simulink model "Joystick"  (R2023b)
settings: Solver=FixedStepAuto  StartTime=0.0  StopTime=t_Total  FixedStep=dt  RelTol=1e-3
undefined symbols (not defined in the file): delta_E_max, delta_E_min, delta_R_max, delta_R_min, dt
libraries: aerolibanimutils x2
settings Model: Creator=iwl  LastModifiedBy=iwl
settings ModelReferenceCC: EnableRefExpFcnMdlSchedulingChecks=on

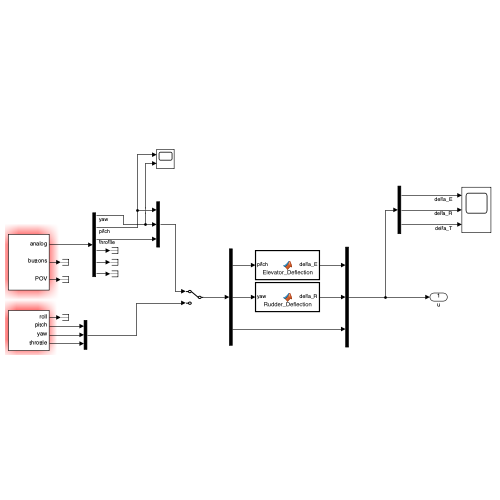
[thumbnail: Simulink's stored preview of the top-level diagram]
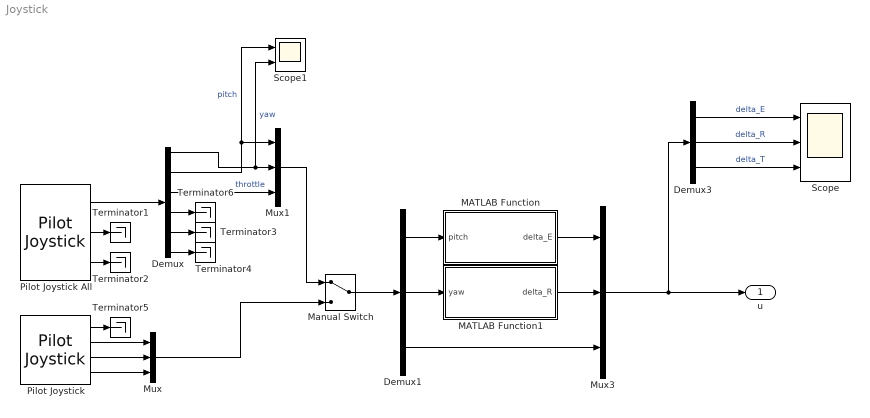
== system Joystick ==
  Demux : Demux  Outputs=6
  Demux1 : Demux  Outputs=3
  Demux3 : Demux  Outputs=3
  MATLAB Function : MATLAB Function  TreatAsAtomicUnit=on
  MATLAB Function1 : MATLAB Function  TreatAsAtomicUnit=on
  Manual Switch : ManualSwitch
  Mux : Mux  Inputs=3
  Mux1 : Mux  Inputs=3
  Mux3 : Mux  Inputs=3
  Pilot Joystick : aerolibanimutils/Pilot Joystick  JoystickID=Joystick1  OutputConfiguration=FourAxis  SampleTime=dt
  Pilot Joystick All : aerolibanimutils/Pilot Joystick  JoystickID=Joystick1  OutputConfiguration=AllOutputs  SampleTime=dt
  Scope : Scope  NumInputPorts=3
  Scope1 : Scope  NumInputPorts=2
  Terminator{1..6} (6 alike) : Terminator
  u : Outport
  wires:
  Pilot Joystick/1 -> Terminator5/1
  Demux/1 -> Scope1/2, Mux1/2  "yaw"
  Demux/5 -> Terminator3/1
  Mux1/1 -> Manual Switch/1
  Pilot Joystick All/1 -> Demux/1
  Mux/1 -> Manual Switch/2
  Demux1/3 -> Mux3/3
  Pilot Joystick All/2 -> Terminator1/1
  Pilot Joystick/2 -> Mux/1
  Pilot Joystick All/3 -> Terminator2/1
  Demux/2 -> Scope1/1, Mux1/1  "pitch"
  Pilot Joystick/3 -> Mux/2
  Pilot Joystick/4 -> Mux/3
  Demux/3 -> Mux1/3  "throttle"
  Demux/6 -> Terminator4/1
  Mux3/1 -> Demux3/1, u/1
  Demux3/2 -> Scope/2  "delta_R"
  Demux3/1 -> Scope/1  "delta_E"
  Demux3/3 -> Scope/3  "delta_T"
  Demux/4 -> Terminator6/1
  Manual Switch/1 -> Demux1/1
  MATLAB Function1/1(delta_R) -> Mux3/2
  Demux1/2 -> MATLAB Function1/1(yaw)
  MATLAB Function/1(delta_E) -> Mux3/1
  Demux1/1 -> MATLAB Function/1(pitch)

== matlab function Joystick/MATLAB Function ==
  data: pitch input; delta_E output; delta_E_min parameter; delta_E_max parameter
function delta_E = Elevator_Deflection(pitch, delta_E_min, delta_E_max)
    
    if pitch >= 0
        delta_E = pitch * delta_E_max;
    else
        delta_E = pitch * delta_E_min;
    end
    
end

== matlab function Joystick/MATLAB Function1 ==
  data: yaw input; delta_R_min parameter; delta_R output; delta_R_max parameter
function delta_R = Rudder_Deflection(yaw, delta_R_min, delta_R_max)
    
    if yaw >= 0
        delta_R = yaw * delta_R_max;
    else
        delta_R = yaw * delta_R_min;
    
end
